simulink model "aufgabe_6_sim"  (R2016b)
settings: Solver=VariableStepAuto  StartTime=0.0  StopTime=14  RelTol=1e-3
values from neighbouring files (symbols this model uses):
  A_lin = [ -R_GSM/L_GSM, 0, -k_GSM/L_GSM, 0;      0, 0, 1, -1;      k_GSM/J_GSM, -c_GSMP/J_GSM, -(d_GSMP + d_vGSM)/J_GSM, d_GSMP/J_GSM;      0, c_GSMP/J_P, d_GSMP/J_P, -(d_GSMP + d_vP + 2*d_qP*w_P_r)/J_P]    [aufgabe_4.m]    (also in aufgabe_6.m)
  A_red = [0,1,-1;  -c_GSMP/J_GSM, -(k_GSM^2/R_GSM + d_GSMP + d_vGSM)/J_GSM, d_GSMP/J_GSM;  c_GSMP/J_P, d_GSMP/J_P, -(d_GSMP + d_vP + 2*d_qP*w_P_r_red)/J_P]    [aufgabe_4.m]    (also in aufgabe_6.m)
  b_lin = [bu_lin bd_lin]    [aufgabe_4.m]    (also in aufgabe_6.m)
  b_red = [bu_red bd_red]    [aufgabe_4.m]    (also in aufgabe_6.m)
  i_GSM_r = (u_GSM_r + (k_GSM*(R_GSM*d_vP + R_GSM*d_vGSM -      (k_GSM^4 + R_GSM^2*d_vP^2 + R_GSM^2*d_vGSM^2 -      4*M_ext_r*R_GSM^2*d_qP - 4*R_GSM^2*d_cP*d_qP -      4*R_GSM^2*d_cGSM*d_qP + 2*R_GSM^2*d_vP*d_vGSM +      2*R_GSM*d_vP*k_GSM^2 + 2*R_GSM*d_vGSM*k_GSM^2 +      4*R_GSM*d_qP*k_GSM*u_GSM_r)^(1/2) + k_GSM^2))/(2*R_GSM*d_qP))/R_GSM    [aufgabe_4.m]    (also in aufgabe_6.m)
  k_GSM = block.DialogPrm(3).Data    [GSMP_S_m.m]    (also in aufgabe_4.m = 0.1; aufgabe_6.m = 0.1)
  M_ext_r = 0    [aufgabe_4.m]    (also in aufgabe_6.m)
  phi_GSMP_r = ((k_GSM^2 + R_GSM*d_vGSM)*(R_GSM*d_vP + R_GSM*d_vGSM -      (k_GSM^4 + R_GSM^2*d_vP^2 + R_GSM^2*d_vGSM^2 -      4*M_ext_r*R_GSM^2*d_qP - 4*R_GSM^2*d_cP*d_qP -      4*R_GSM^2*d_cGSM*d_qP + 2*R_GSM^2*d_vP*d_vGSM +      2*R_GSM*d_vP*k_GSM^2 + 2*R_GSM*d_vGSM*k_GSM^2 +      4*R_GSM*d_qP*k_GSM*u_GSM_r)^(1/2) + k_GSM^2))/(2*R_GSM^2*c_GSMP*d_qP)     - (R_GSM*d_cGSM - k_GSM*u_GSM_r)/(R_GSM*c_GSMP)    [aufgabe_4.m]    (also in aufgabe_6.m)
  R_GSM = block.DialogPrm(2).Data    [GSMP_S_m.m]    (also in aufgabe_4.m = 0.46; aufgabe_6.m = 0.46)
  u_GSM_r = 5.6    [aufgabe_4.m]    (also in aufgabe_6.m)
  w_GSM_r = -(R_GSM*d_vP + R_GSM*d_vGSM - (k_GSM^4 + R_GSM^2*d_vP^2 +      R_GSM^2*d_vGSM^2 - 4*M_ext_r*R_GSM^2*d_qP -      4*R_GSM^2*d_cP*d_qP - 4*R_GSM^2*d_cGSM*d_qP +      2*R_GSM^2*d_vP*d_vGSM + 2*R_GSM*d_vP*k_GSM^2 +      2*R_GSM*d_vGSM*k_GSM^2 + 4*R_GSM*d_qP*k_GSM*u_GSM_r)^(1/2) +      k_GSM^2)/(2*R_GSM*d_qP)    [aufgabe_4.m]    (also in aufgabe_6.m)
  w_P_r = -(R_GSM*d_vP + R_GSM*d_vGSM - (k_GSM^4 + R_GSM^2*d_vP^2 +      R_GSM^2*d_vGSM^2 - 4*M_ext_r*R_GSM^2*d_qP -      4*R_GSM^2*d_cP*d_qP - 4*R_GSM^2*d_cGSM*d_qP +      2*R_GSM^2*d_vP*d_vGSM + 2*R_GSM*d_vP*k_GSM^2 +      2*R_GSM*d_vGSM*k_GSM^2 + 4*R_GSM*d_qP*k_GSM*u_GSM_r)^(1/2) +      k_GSM^2)/(2*R_GSM*d_qP)    [aufgabe_4.m]    (also in aufgabe_5.m = -(R_GSM*d_vP + R_GSM*d_vGSM - (k_GSM^4 + R_GSM^2*d_vP^2 +   ; aufgabe_6.m)
undefined symbols (not defined in the file): c_GSMP, d_cGSM, d_cP, d_GSMP, d_qP, d_vGSM, d_vP, i_GSM_0, J_GSM, J_P, L_GSM, phi_GSMP_0, w_GSM_0, w_P_0
settings Model: Creator=M  LastModifiedBy=floz

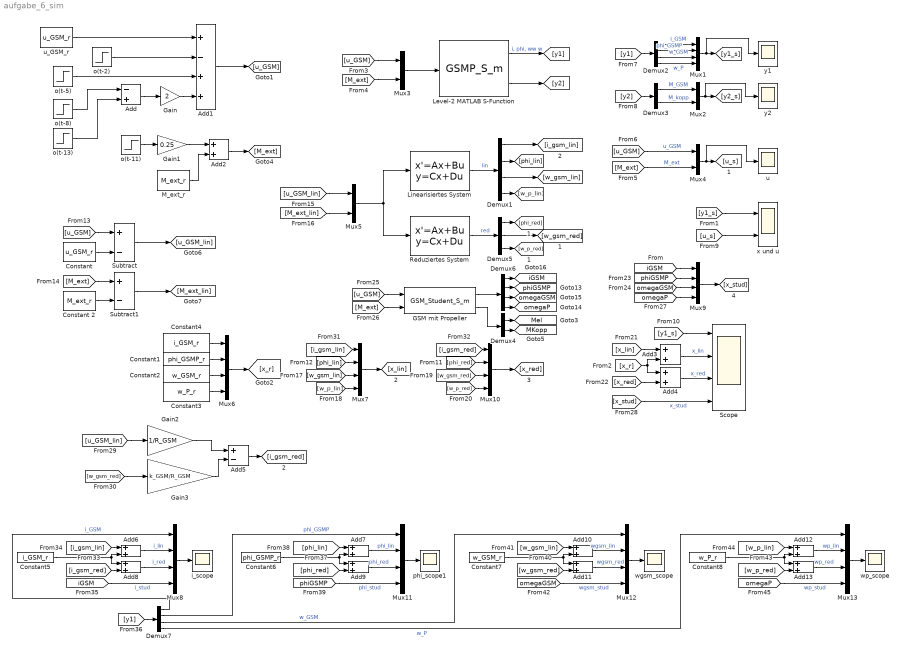
== system aufgabe_6_sim ==
  Add : Sum  Inputs=-+
  Add1 : Sum  Inputs=+-++
  Add{2..4,6..13} (11 alike) : Sum
  Add5 : Sum  Inputs=+-
  Constant : Constant  Value=u_GSM_r
  Constant 2 : Constant  Value=M_ext_r
  Constant1 : Constant  Value=phi_GSMP_r
  Constant2 : Constant  Value=w_GSM_r
  Constant3 : Constant  Value=w_P_r
  Constant4 : Constant  Value=i_GSM_r
  Constant5 : Constant  Value=i_GSM_r
  Constant6 : Constant  Value=phi_GSMP_r
  Constant7 : Constant  Value=w_GSM_r
  Constant8 : Constant  Value=w_P_r
  Demux{1..2,6..7} (4 alike) : Demux
  Demux3 : Demux  Outputs=2
  Demux4 : Demux  Outputs=2
  Demux5 : Demux  Outputs=3
  GSM mit Propeller : M-S-Function  FunctionName=GSM_Student_S_m  Parameters=iGSM_0,phiGSMP_0,omegaGSM_0,omegaP_0  mask{iGSM_0=i_GSM_r, phiGSMP_0=phi_GSMP_r, omegaGSM_0=w_GSM_r, omegaP_0=w_P_r}
      mask prompts: iGSM_0 "Anfangsbedingung iGSM"; phiGSMP_0 "Anfangsbedingung phiGSMP"; omegaGSM_0 "Anfangsbedingung omegaGSM"; omegaP_0 "Anfangsbedingung omegaP"
  Gain : Gain  Gain=2
  Gain1 : Gain  Gain=0.25
  Gain2 : Gain  Gain=1/R_GSM
  Gain3 : Gain  Gain=k_GSM/R_GSM
  Level-2 MATLAB S-Function : M-S-Function  FunctionName=GSMP_S_m  Parameters=L_GSM, R_GSM, k_GSM, J_GSM, d_cGSM, d_vGSM, J_P, d_cP, d_vP, d_qP, c_GSMP, d_GSMP, i_GSM_0, phi_GSMP_0, w_GSM_0, w_P_0  mask{L_GSM=L_GSM, R_GSM=R_GSM, k_GSM=k_GSM, J_GSM=J_GSM, d_cGSM=d_cGSM, d_vGSM=d_vGSM, J_P=J_P, d_cP=d_cP, d_vP=d_vP, d_qP=d_qP, c_GSMP=c_GSMP, d_GSMP=d_GSMP, i_GSM_0=i_GSM_0, phi_GSMP_0=phi_GSMP_0, w_GSM_0=w_GSM_0, w_P_0=w_P_0}
      mask prompts: i_GSM_0 "i_GSM"; phi_GSMP_0 "phi_GSMP"; w_GSM_0 "w_GSM"; w_P_0 "w_P"
      mask DialogControl Container3 Prompt: Anfangszustände
  Linearisiertes System : StateSpace  A=A_lin  B=b_lin  C=[1 0 0 0; 0 1 0 0; 0 0 1 0; 0 0 0 1]  D=[0 0; 0 0; 0 0; 0 0]  X0=0
  M_ext_r : Constant  Value=M_ext_r
  Mux{1,6..13} (9 alike) : Mux
  Mux{2..5} (4 alike) : Mux  Inputs=2
  Reduziertes System : StateSpace  A=A_red  B=b_red  C=[1 0 0; 0 1 0; 0 0 1]  D=[0 0; 0 0; 0 0]  X0=0
  Scope : Scope  NumInputPorts=4
  Subtract : Sum  Inputs=+-
  Subtract1 : Sum  Inputs=+-
  i_scope : Scope
  o(t-11) : Step  Time=11  SampleTime=0
  o(t-13) : Step  Time=13  SampleTime=0
  o(t-2) : Step  Time=2  SampleTime=0
  o(t-5) : Step  Time=5  SampleTime=0
  o(t-8) : Step  Time=8  SampleTime=0
  phi_scope1 : Scope
  u : Scope
  "u_GSM_r " : Constant  Value=u_GSM_r
  wgsm_scope : Scope
  wp_scope : Scope
  x und u : Scope  NumInputPorts=2
  "y1 " : Scope
  "y2 " : Scope
  tag scope: MKopp=global, Mel=global, iGSM=global, omegaGSM=global, omegaP=global, phiGSMP=global
  wires:
  Mux3/1 -> Level-2 MATLAB S-Function/1
  [u_GSM] -> Mux3/1
  [M_ext] -> Mux3/2
  Level-2 MATLAB S-Function/1 -> [y1]  "i, phi, ww w"
  Level-2 MATLAB S-Function/2 -> [y2]
  "u_GSM_r "/1 -> Add1/1
  Add1/1 -> [u_GSM]
  o(t-2)/1 -> Add1/2
  o(t-8)/1 -> Add/1
  o(t-13)/1 -> Add/2
  Add/1 -> Gain/1
  o(t-5)/1 -> Add1/3
  Gain/1 -> Add1/4
  Gain1/1 -> Add2/1
  M_ext_r/1 -> Add2/2
  o(t-11)/1 -> Gain1/1
  Add2/1 -> [M_ext]
  [y1] -> Demux2/1
  Demux2/1 -> Mux1/1  "i_GSM"
  Demux2/2 -> Mux1/2  "phi_GSMP"
  Demux2/3 -> Mux1/3  "w_GSM"
  Demux2/4 -> Mux1/4  "w_P"
  Mux1/1 -> "y1 "/1, [y1_s]
  Demux3/2 -> Mux2/2  "M_kopp"
  [y2] -> Demux3/1
  Demux3/1 -> Mux2/1  "M_GSM"
  Mux2/1 -> "y2 "/1, [y2_s]
  [u_GSM] -> Mux4/1  "u_GSM"
  [M_ext] -> Mux4/2  "M_ext"
  Mux4/1 -> u/1, [u_s]
  [y1_s] -> x und u/1
  [u_s] -> x und u/2
  Mux5/1 -> Reduziertes System/1, Linearisiertes System/1
  Subtract/1 -> [u_GSM_lin]
  Constant/1 -> Subtract/2
  [u_GSM] -> Subtract/1
  Subtract1/1 -> [M_ext_lin]
  Constant 2/1 -> Subtract1/2
  [M_ext] -> Subtract1/1
  [M_ext_lin] -> Mux5/2
  [u_GSM_lin] -> Mux5/1
  Linearisiertes System/1 -> Demux1/1  "lin"
  Reduziertes System/1 -> Demux5/1  "red"
  Demux5/1 -> [phi_red]
  Demux5/3 -> [w_p_red]
  Constant3/1 -> Mux6/4
  Mux6/1 -> [x_r]
  [x_r] -> Add3/2, Add4/1
  Add3/1 -> Scope/2  "x_lin"
  [y1_s] -> Scope/1
  [phi_lin] -> Mux7/2
  [w_gsm_lin] -> Mux7/3
  [w_p_lin] -> Mux7/4
  Mux7/1 -> [x_lin]
  [x_lin] -> Add3/1
  [x_red] -> Add4/2
  Demux5/2 -> [w_gsm_red]
  [u_GSM] -> GSM mit Propeller/1
  [M_ext] -> GSM mit Propeller/2
  Demux6/1 -> [iGSM]
  Demux6/2 -> [phiGSMP]
  Demux6/3 -> [omegaGSM]
  Demux6/4 -> [omegaP]
  GSM mit Propeller/1 -> Demux6/1
  GSM mit Propeller/2 -> Demux4/1
  Demux4/1 -> [Mel]
  Demux4/2 -> [MKopp]
  [iGSM] -> Mux9/1
  [phiGSMP] -> Mux9/2
  [omegaGSM] -> Mux9/3
  [omegaP] -> Mux9/4
  Mux9/1 -> [x_stud]
  [x_stud] -> Scope/4  "x_stud"
  Demux1/4 -> [w_p_lin]
  Demux1/3 -> [w_gsm_lin]
  Demux1/2 -> [phi_lin]
  Demux1/1 -> [i_gsm_lin]
  [u_GSM_lin] -> Gain2/1
  [w_gsm_red] -> Gain3/1
  Add5/1 -> [i_gsm_red]
  Gain2/1 -> Add5/1
  Gain3/1 -> Add5/2
  [i_gsm_lin] -> Mux7/1
  [i_gsm_red] -> Mux10/1
  [phi_red] -> Mux10/2
  [w_gsm_red] -> Mux10/3
  [w_p_red] -> Mux10/4
  Mux10/1 -> [x_red]
  Constant1/1 -> Mux6/2
  Constant2/1 -> Mux6/3
  Constant4/1 -> Mux6/1
  Add4/1 -> Scope/3  "x_red"
  [iGSM] -> Mux8/4  "i_stud"
  [i_gsm_lin] -> Add6/1
  [i_gsm_red] -> Add8/2
  Add8/1 -> Mux8/3  "i_red"
  Add6/1 -> Mux8/2  "i_lin"
  Constant5/1 -> Add8/1, Add6/2
  [y1] -> Demux7/1
  Demux7/1 -> Mux8/1  "i_GSM"
  Demux7/2 -> Mux11/1  "phi_GSMP"
  Demux7/3 -> Mux12/1  "w_GSM"
  Demux7/4 -> Mux13/1  "w_P"
  Mux8/1 -> i_scope/1
  [phiGSMP] -> Mux11/4  "phi_stud"
  [phi_lin] -> Add7/1
  [phi_red] -> Add9/2
  Add9/1 -> Mux11/3  "phi_red"
  Add7/1 -> Mux11/2  "phi_lin"
  Constant6/1 -> Add9/1, Add7/2
  Mux11/1 -> phi_scope1/1
  [omegaGSM] -> Mux12/4  "wgsm_stud"
  [w_gsm_lin] -> Add10/1
  [w_gsm_red] -> Add11/2
  Add11/1 -> Mux12/3  "wgsm_red"
  Add10/1 -> Mux12/2  "wgsm_lin"
  Constant7/1 -> Add11/1, Add10/2
  Mux12/1 -> wgsm_scope/1
  [omegaP] -> Mux13/4  "wp_stud"
  [w_p_lin] -> Add12/1
  [w_p_red] -> Add13/2
  Add13/1 -> Mux13/3  "wp_red"
  Add12/1 -> Mux13/2  "wp_lin"
  Constant8/1 -> Add13/1, Add12/2
  Mux13/1 -> wp_scope/1
